simulink subsystem "Axial_Drag"  (R2025b)
settings: Solver=VariableStepAuto  StartTime=0.0  StopTime=10.0  RelTol=1e-3
undefined symbols (not defined in the file): body_length, CD_data, CD_input, drag_factor, rocket_area_frontal, rocket_diameter
libraries: aerolibasang x2
settings Model: Creator=joedo  LastModifiedBy=finnb

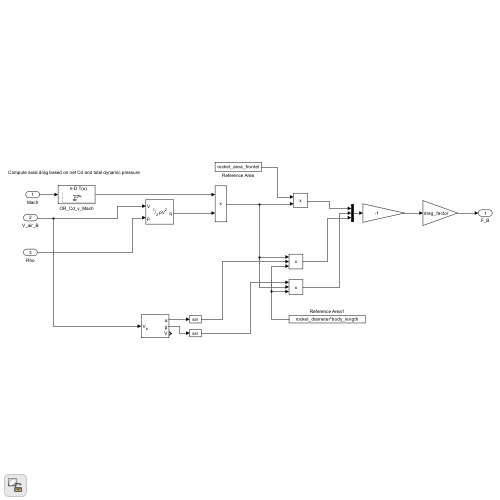
[thumbnail: Simulink's stored preview of the top-level diagram]
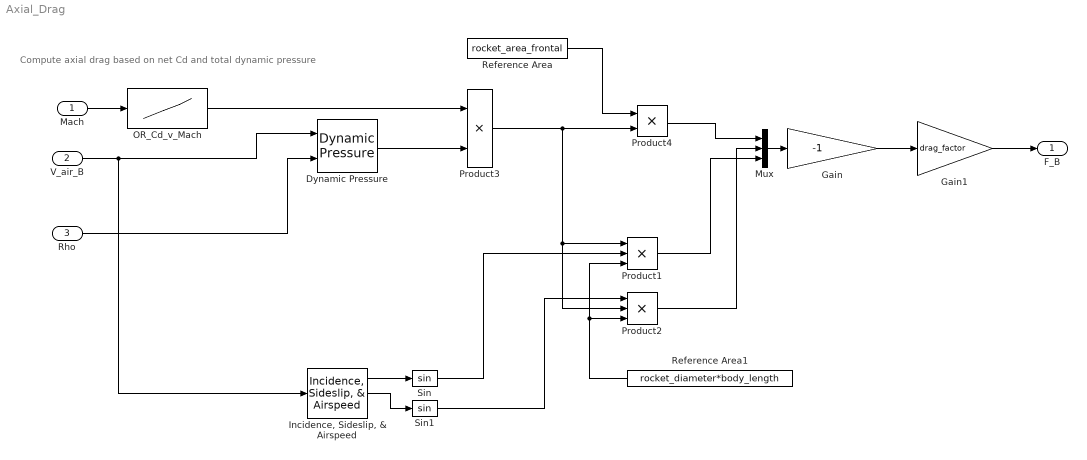
== system Axial_Drag ==
  note: Compute axial drag based on net Cd and total dynamic pressure
  Mach : Inport
  V_air_B : Inport  Port=2
  Rho : Inport  Port=3
  Dynamic Pressure : aerolibasang/Dynamic Pressure
  Gain : Gain  Gain=-1
  Gain1 : Gain  Gain=drag_factor
  "Incidence, Sideslip, & Airspeed" : aerolibasang/Incidence, Sideslip, & Airspeed
  Mux : Mux  Inputs=3
  OR_Cd_v_Mach : Lookup_n-D  NumberOfTableDimensions=1  BreakpointsForDimension1=CD_input  Table=CD_data  InternalRulePriority=Speed  RndMeth=Simplest
  Product1 : Product  Inputs=3
  Product2 : Product  Inputs=3
  Product3 : Product
  Product4 : Product
  Reference Area : Constant  Value=rocket_area_frontal
  Reference Area1 : Constant  Value=rocket_diameter*body_length
  Sin : Trigonometry
  Sin1 : Trigonometry
  F_B : Outport  VectorParamsAs1DForOutWhenUnconnected=off
  wires:
  Mach/1 -> OR_Cd_v_Mach/1
  OR_Cd_v_Mach/1 -> Product3/1
  Gain1/1 -> F_B/1
  Gain/1 -> Gain1/1
  V_air_B/1 -> "Incidence, Sideslip, & Airspeed"/1, Dynamic Pressure/1
  Rho/1 -> Dynamic Pressure/2
  Reference Area/1 -> Product4/1
  Reference Area1/1 -> Product1/3, Product2/3
  "Incidence, Sideslip, & Airspeed"/1 -> Sin/1
  "Incidence, Sideslip, & Airspeed"/2 -> Sin1/1
  Sin1/1 -> Product2/1
  Sin/1 -> Product1/2
  Product3/1 -> Product2/2, Product1/1, Product4/2
  Mux/1 -> Gain/1
  Product1/1 -> Mux/3
  Product2/1 -> Mux/2
  Dynamic Pressure/1 -> Product3/2
  Product4/1 -> Mux/1
